simulink model "dynamic_model_dab"  (R2022b)
settings: Solver=VariableStepAuto  StartTime=0.0  StopTime=6.5e-2  RelTol=1e-3
libraries: spsMosfetLib x8, spsSeriesRLCBranchLib x5, spsEdgeDetectorLib x4, spsCurrentMeasurementLib x3, spsStairGeneratorLib x3, spsControlledVoltageSourceLib x2, spsMultimeterLib x2, spsLinearTransformerLib x1, eeGeneralControl x1, spsMeanVariableFrequencyLib x1, spsMeanLib x1, slpidlib x1
settings Model: Creator=srikr  LastModifiedBy=Pratik

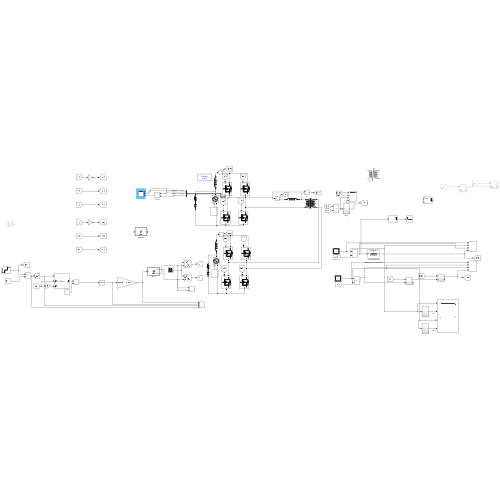
[thumbnail: Simulink's stored preview of the top-level diagram]
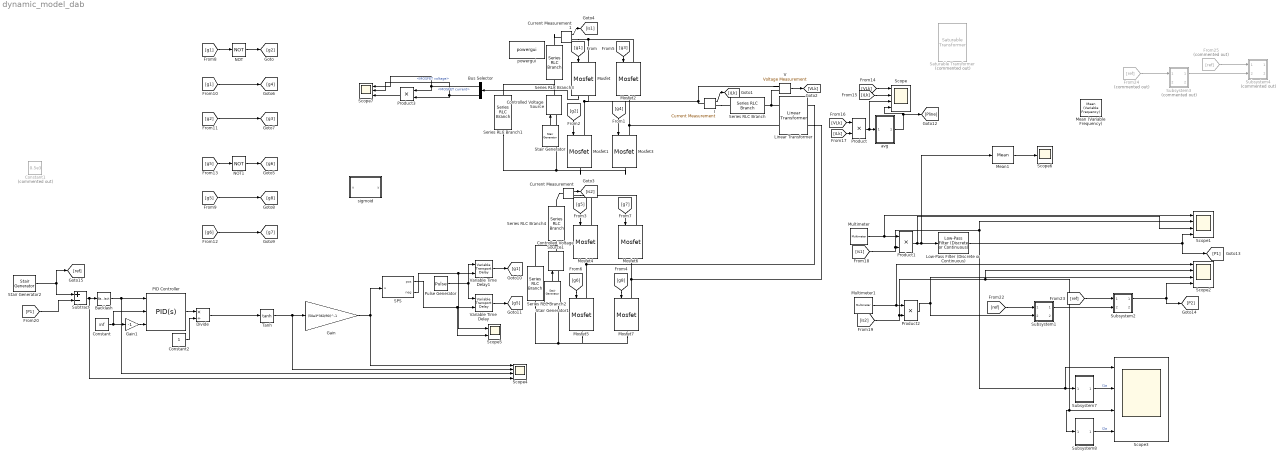
== system dynamic_model_dab ==
  Backlash : Backlash  BacklashWidth=0
  Bus Selector : BusSelector  OutputSignals=MOSFET current,MOSFET voltage
  Constant : Constant  Value=inf
  Constant1 : Constant  Commented=on  Value=0.5e3
  Constant2 : Constant
  Controlled Voltage Source : spsControlledVoltageSourceLib/Controlled Voltage Source  Initialize=on  Source_Type=AC  Amplitude=0  Phase=0  Frequency=0  Measurements=Voltage
  Controlled Voltage Source1 : spsControlledVoltageSourceLib/Controlled Voltage Source  Initialize=on  Source_Type=AC  Amplitude=0  Phase=0  Frequency=0  Measurements=Voltage
  Current Measurement : spsCurrentMeasurementLib/Current Measurement  PhasorSimulation=off  OutputType=Complex  PSBequivalent=0
  Current Measurement1 : spsCurrentMeasurementLib/Current Measurement  PhasorSimulation=off  OutputType=Complex  PSBequivalent=0
  Divide : Product  Inputs=*/
  From24 : From  Commented=on  GotoTag=ref
  From25 : From  Commented=on  GotoTag=ref
  Gain : Gain  Gain=(50e3*360/90)^-1
  Gain1 : Gain  Gain=-1
  I : spsCurrentMeasurementLib/Current Measurement  PhasorSimulation=off  OutputType=Complex  PSBequivalent=0
  Linear Transformer : spsLinearTransformerLib/Linear Transformer  UNITS=SI  NominalPower=[ 250e6 30e3 ]  winding1=[200 0 0]  winding2=[100 0 0]  ThreeWindings=off  winding3=[3.15e+05 0.7938 0.084225]  RmLm=[30e3 1e-3]  Measurements=All voltages and currents  DataType=on
  Low-Pass Filter (Discrete or Continuous) : eeGeneralControl/Low-Pass Filter (Discrete or Continuous)  K=1  T=1e-3  B=inf  A=-inf  init_option=Inherited from block input  x0=0  Ts=-1
  Mean (Variable Frequency) : spsMeanVariableFrequencyLib/Mean (Variable Frequency)  Finit=60  Fmin=45  Vinit=0  Ts=0
      settings: LibrarySourceBlock=|
      | sps_lib/Sensors and Measurements/Mean
      | (Variable Frequency)
  Mean1 : spsMeanLib/Mean  Freq=50e3  Vinit=0  Ts=0
  Mosfet : spsMosfetLib/Mosfet  Ron=0.1  Lon=0  Rd=0.01  Vfd=0  IC=0  Rs=1e5  Cs=inf  Measurements=on
  Mosfet{1..7} (7 alike) : spsMosfetLib/Mosfet  Ron=0.1  Lon=0  Rd=0.01  Vfd=0  IC=0  Rs=1e5  Cs=inf  Measurements=off
  Multimeter : spsMultimeterLib/Multimeter  L=11  sel=4  yselected={}  Gain=1  OutputType=Complex  PlotAtSimulationStop=off  PhasorSimulation=off
  Multimeter1 : spsMultimeterLib/Multimeter  L=11  sel=4  yselected={}  Gain=1  OutputType=Complex  PlotAtSimulationStop=off  PhasorSimulation=off
  NOT : Logic  Operator=NOT  IconShape=distinctive  AllPortsSameDT=off  OutDataTypeStr=boolean
  NOT1 : Logic  Operator=NOT  IconShape=distinctive  AllPortsSameDT=off  OutDataTypeStr=boolean
  PID Controller : slpidlib/PID Controller  Controller=PID  Form=Parallel  TimeDomain=Continuous-time  UseExternalTs=off  SampleTime=-1  IntegratorMethod=Forward Euler  FilterMethod=Forward Euler  ControllerParametersSource=internal  P=9e-2  I=0  UseKiTs=off  D=0  N=100  UseFilter=on  TunerSelectOption=Transfer Function Based (PID Tuner App)  InitialConditionSource=internal  InitialConditionForIntegrator=0  InitialConditionForFilter=0  DifferentiatorICPrevScaledInput=0  ExternalReset=none  TrackingMode=off  Kt=1  LimitOutput=on  SatLimitsSource=external  UpperSaturationLimit=1e3  LowerSaturationLimit=-1e3  LinearizeAsGain=on  AntiWindupMode=none  Kb=1  LimitIntegrator=off  UpperIntegratorSaturationLimit=inf  LowerIntegratorSaturationLimit=-inf  POutMin=[]  POutMax=[]  IOutMin=[]  IOutMax=[]  DOutMin=[]  DOutMax=[]  NOutMin=[]  NOutMax=[]  SumOutMin=[]  SumOutMax=[]  SaturationOutMin=[]  SaturationOutMax=[]  PParamMin=[]  PParamMax=[]  IParamMin=[]  IParamMax=[]  DParamMin=[]  DParamMax=[]  NParamMin=[]  NParamMax=[]  KbParamMin=[]  KbParamMax=[]  KtParamMin=[]  KtParamMax=[]  KbOutMin=[]  KbOutMax=[]  KtOutMin=[]  KtOutMax=[]  IntegratorOutMin=[]  IntegratorOutMax=[]  FilterOutMin=[]  FilterOutMax=[]  SumI1OutMin=[]  SumI1OutMax=[]  SumI2OutMin=[]  SumI2OutMax=[]  SumI3OutMin=[]  SumI3OutMax=[]  SumI4OutMin=[]  SumI4OutMax=[]  SumDOutMin=[]  SumDOutMax=[]  DifferentiatorOutMin=[]  DifferentiatorOutMax=[]  FilterDiffOutCoefMin=[]  FilterDiffOutCoefMax=[]  ReciprocalOutMin=[]  ReciprocalOutMax=[]  SumDenOutMin=[]  SumDenOutMax=[]  SumNumOutMin=[]  SumNumOutMax=[]  DivideOutMin=[]  DivideOutMax=[]  UdiffTsProdOutMin=[]  UdiffTsProdOutMax=[]  NTsProdOutMin=[]  NTsProdOutMax=[]  UintegralTsProdOutMin=[]  UintegralTsProdOutMax=[]  UngainTsProdOutMin=[]  UngainTsProdOutMax=[]  ClampingZeroOutDataTypeStr=Inherit: Inherit via back propagation  ClampingZeroOutMin=[]  ClampingZeroOutMax=[]  FilterDenConstantOutDataTypeStr=Inherit: Inherit via back propagation  FilterDenConstantOutMin=[]  FilterDenConstantOutMax=[]  PCopyOutDataTypeStr=Inherit: Inherit via back propagation  PCopyOutMin=[]  PCopyOutMax=[]  NCopyOutDataTypeStr=Inherit: Inherit via back propagation  NCopyOutMin=[]  NCopyOutMax=[]  IntegratorContinuousStateAttributes=''  IntegratorStateMustResolveToSignalObject=off  IntegratorRTWStateStorageClass=Auto  FilterContinuousStateAttributes=''  FilterStateMustResolveToSignalObject=off  FilterRTWStateStorageClass=Auto  ParallelPVariant=InternalParameters  IdealPVariant=Disabled  IVariant=InternalParameters  DVariant=InternalParameters  IntegratorVariant=Continuous  SatVariant=External  AWVariant=Passthrough  PCopyVariant=Disabled  TRVariant=Disabled  FdbkBlocksVariant=Forward  IdealPFdbkVariant=Disabled  SatFdbkVariant=Disabled  DerivativeFilterVariant=ContFilter  NVariant=InternalParameters  NCopyVariant=Disabled  FilterICVariant=InternalICsFilter  IntegratorICVariant=InternalICs  ExternalResetVariant=Disabled  TRSumVariant=Passthrough  SumFdbkVariant=Disabled  SumVariant=Sum_PID  TsampFilterVariant=InternalTs  TsampNgainVariant=Passthrough  TsampIntegralVariant=Passthrough  ExternalSaturationOutDataTypeStr=Inherit: Same as second input
  Product{,1..3} (4 alike) : Product
  Pulse Generator : DiscretePulseGenerator  PulseType=Time based  Period=1/50e3  PulseWidth=50
  SPS : MATLAB Function  TreatAsAtomicUnit=on
  Saturable Transformer : spsSaturableTransformerLib/Saturable Transformer  Commented=on  ThreeWindings=off  Hysteresis=off  DataFile='hysteresis.mat'  Measurements=All measurements (V I Flux)  UNITS=SI  NominalPower=[250e6 60]  Winding1=[200 0 0]  Winding2=[100 0 0]  Winding3=[3.15e+05 0.7938 0.084225]  Saturation=[0 0;1 100;]  CoreLoss=25e3  BreakLoop=off  DiscreteSolver=Trapezoidal iterative  DataType=on  InitialFlux=0  TransfoNumber=1
      settings: LibrarySourceBlock=sps_lib/Power Grid Elements/Saturable Transformer
  Scope{,1..4} (5 alike) : Scope  NumInputPorts=4
  Scope5 : Scope  NumInputPorts=2
  Scope6 : Scope
  Scope7 : Scope  NumInputPorts=3
  Series RLC Branch : spsSeriesRLCBranchLib/Series RLC Branch  LConnTagsString=__new0  RConnTagsString=__new0  BranchType=L  Resistance=1  Inductance=10e-6  SetiL0=off  InitialCurrent=0  Capacitance=1e-6  Setx0=off  InitialVoltage=0  Measurements=Branch voltage and current
  Series RLC Branch1 : spsSeriesRLCBranchLib/Series RLC Branch  LConnTagsString=__new0  RConnTagsString=__new0  BranchType=RC  Resistance=1e-9  Inductance=1e-3  SetiL0=off  InitialCurrent=0  Capacitance=1e-6  Setx0=off  InitialVoltage=0  Measurements=None
  Series RLC Branch2 : spsSeriesRLCBranchLib/Series RLC Branch  LConnTagsString=__new0  RConnTagsString=__new0  BranchType=RC  Resistance=1e-9  Inductance=1e-3  SetiL0=off  InitialCurrent=0  Capacitance=1e-6  Setx0=off  InitialVoltage=0  Measurements=None
  Series RLC Branch3 : spsSeriesRLCBranchLib/Series RLC Branch  LConnTagsString=__new0  RConnTagsString=__new0  BranchType=L  Resistance=1e-9  Inductance=2e-6  SetiL0=off  InitialCurrent=0  Capacitance=1e-9  Setx0=off  InitialVoltage=0  Measurements=None
  Series RLC Branch4 : spsSeriesRLCBranchLib/Series RLC Branch  LConnTagsString=__new0  RConnTagsString=__new0  BranchType=L  Resistance=1e-9  Inductance=2e-6  SetiL0=off  InitialCurrent=0  Capacitance=1e-9  Setx0=off  InitialVoltage=0  Measurements=None
  Stair Generator : spsStairGeneratorLib/Stair Generator  t=[0,0.5]*5e-2  e=[100, 100]  Ts=0
  Stair Generator1 : spsStairGeneratorLib/Stair Generator  t=[0,0.25]*5e-2  e=[100, 100]  Ts=0
  Stair Generator2 : spsStairGeneratorLib/Stair Generator  t=[0:.25:1]*5e-2  e=[0.5e3,-1e3,-0e3,1e3,0.5e3]  Ts=0
  Subsystem1 : Subsystem
  Subsystem2 : Subsystem
  Subsystem3 : Subsystem  Commented=on
  Subsystem4 : Subsystem  Commented=on
  Subsystem7 : Subsystem
  Subsystem8 : Subsystem
  Subtract : Sum  Inputs=+-
  Tanh : Trigonometry  Operator=tanh
  V : spsVoltageMeasurementLib/Voltage Measurement  PhasorSimulation=off  OutputType=Complex  PSBequivalent=0
  Variable Time Delay : VariableTransportDelay  MaximumDelay=10
  Variable Time Delay1 : VariableTransportDelay  MaximumDelay=10
  avg : Subsystem
  powergui : sps_lib/powergui  Priority=1  SimulationMode=Discrete  SampleTime=1e-6  frequency=60  Iterations=50  frequencyindice=0  Pbase=100e6  ErrMax=1e-4  UnitsV=kV  UnitsW=MW  buscounter=0  FunctionMessages=off  echomessages=off  EnableUseOfTLC=off  CurrentSourceSwitches=off  DisableSnubberDevices=off  DisableRonSwitches=off  DisableVfSwitches=off  DisplayEquations=off  AutomaticDiscreteSolvers=off  SolverType=Tustin/Backward Euler (TBE)  Interpol=off  ExternalGateDelay=off  methode=off  Ts=100  x0status=blocks  SPID=on  SwTol=0  HookPort=off  NonlinearTolerance=1e-4  nMaxIteration=100  ContinueOnMaxIteration=off  RestoreLinks=warning  ResistiveCurrentMeasurement=off  Frange=[0:2:500]  Ylog=off  Xlog=on  ShowGrid=off  save=off  variable=ZData  structure=0  ZoomFFT=off  StartTime=0.0  cycles=1  DisplayStyle=1  fundamental=60  FreqAxis=off  MaxFrequency=1000  frequencyindicesteady=1  RmsSteady=1  display=off
  sigmoid : MATLAB Function  TreatAsAtomicUnit=on
  wires:
  [g8] -> Mosfet7/1
  [g1] -> NOT/1
  NOT/1 -> [g2]
  [g1] -> [g4]
  [g2] -> [g3]
  [g5] -> NOT1/1
  [g5] -> [g8]
  [g6] -> [g7]
  NOT1/1 -> [g6]
  Pulse Generator/1 -> Variable Time Delay1/1, Variable Time Delay/1
  Variable Time Delay/1 -> [g5]
  Gain/1 -> SPS/1(u), Scope4/1
  I/1 -> [iLk]
  V/1 -> [VLk]
  [VLk] -> Scope/1
  [iLk] -> Scope/2
  Product/1 -> Scope/3, avg/1(In1)
  [VLk] -> Product/1
  [iLk] -> Product/2
  avg/1(Out1) -> [Pline], Scope/4
  Current Measurement/1 -> [is2]
  Multimeter/1 -> Product1/1, Scope1/1
  [is1] -> Scope3/1, Subsystem7/1(In1), Scope1/2, Product1/2
  Current Measurement1/1 -> [is1]
  [is2] -> Subsystem8/1(In1), Scope3/3, Scope2/2, Product2/2
  Multimeter1/1 -> Product2/1, Scope2/1
  Stair Generator/1 -> Controlled Voltage Source/1
  Subsystem7/1(Out1) -> Scope3/2  "I1a"
  Subsystem8/1(Out1) -> Scope3/4  "I2a"
  Stair Generator1/1 -> Controlled Voltage Source1/1
  Subtract/1 -> Scope4/4, Backlash/1
  Stair Generator2/1 -> Subtract/1, [ref]
  [P1] -> Subtract/2
  Subsystem2/1(Out1) -> [P2], Scope2/4
  Variable Time Delay1/1 -> [g1]
  Backlash/1 -> Scope4/3, PID Controller/1
  Constant/1 -> PID Controller/2, Gain1/1
  Gain1/1 -> PID Controller/3
  PID Controller/1 -> Divide/1
  Constant2/1 -> Divide/2
  Tanh/1 -> Gain/1, Scope4/2
  Product2/1 -> Scope2/3, Subsystem1/2(In2)
  [ref] -> Subsystem1/1(In1)
  Subsystem1/1(Out1) -> Subsystem2/2(In2)
  [ref] -> Subsystem2/1(In1)
  Subsystem3/1(Out1) -> Subsystem4/2(In2)
  From25/1 -> Subsystem4/1(In1)
  From24/1 -> Subsystem3/1(In1)
  Product1/1 -> Low-Pass Filter (Discrete or Continuous)/1, Mean1/1, Scope1/3
  SPS/1(pos) -> Scope5/2, Variable Time Delay/2
  SPS/2(neg) -> Scope5/1, Variable Time Delay1/2
  Mean1/1 -> Scope6/1
  Low-Pass Filter (Discrete or Continuous)/1 -> [P1], Scope1/4
  [g1] -> Mosfet/1
  [g2] -> Mosfet1/1
  [g4] -> Mosfet3/1
  [g3] -> Mosfet2/1
  [g5] -> Mosfet4/1
  [g6] -> Mosfet5/1
  [g7] -> Mosfet6/1
  Divide/1 -> Tanh/1
  Bus Selector/1 -> Scope7/1, Product3/1  "<MOSFET current>"
  Mosfet/1 -> Bus Selector/1
  Bus Selector/2 -> Scope7/2, Product3/2  "<MOSFET voltage>"
  Product3/1 -> Scope7/3
  connections:
  Current Measurement1/RConn1 -- Mosfet/LConn1 -- Mosfet2/LConn1
  Series RLC Branch1/RConn1 -- Controlled Voltage Source/LConn1 -- Mosfet3/RConn1 -- Mosfet1/RConn1
  Series RLC Branch2/RConn1 -- Mosfet7/RConn1 -- Mosfet5/RConn1 -- Controlled Voltage Source1/LConn1
  Current Measurement/RConn1 -- Mosfet4/LConn1 -- Mosfet6/LConn1
  Series RLC Branch/RConn1 -- V/LConn2 -- Linear Transformer/LConn1
  I/RConn1 -- Series RLC Branch/LConn1
  Controlled Voltage Source/RConn1 -- Series RLC Branch1/LConn1 -- Series RLC Branch3/RConn1
  Series RLC Branch4/LConn1 -- Current Measurement/LConn1
  I/LConn1 -- V/LConn1 -- Mosfet1/LConn1 -- Mosfet/RConn1
  Mosfet3/LConn1 -- Mosfet2/RConn1 -- Linear Transformer/LConn2
  Mosfet4/RConn1 -- Linear Transformer/RConn1 -- Mosfet5/LConn1
  Mosfet7/LConn1 -- Mosfet6/RConn1 -- Linear Transformer/RConn2
  Series RLC Branch3/LConn1 -- Current Measurement1/LConn1
  Controlled Voltage Source1/RConn1 -- Series RLC Branch2/LConn1 -- Series RLC Branch4/RConn1

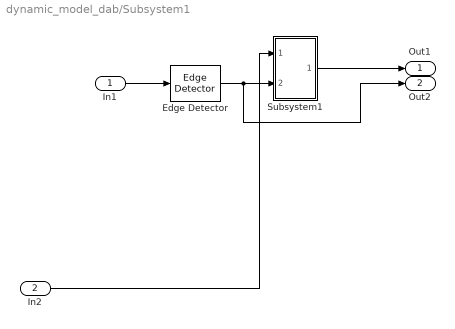
== system dynamic_model_dab/Subsystem1 ==
  In1 : Inport
  In2 : Inport  Port=2
  Edge Detector : spsEdgeDetectorLib/Edge Detector  model=Either  ic=0  Ts=0
      settings: LibrarySourceBlock=sps_lib/Control/Edge Detector
  Subsystem1 : Subsystem
  Out1 : Outport
  Out2 : Outport  Port=2
  wires:
  Edge Detector/1 -> Out2/1, Subsystem1/2(Input)
  Subsystem1/1(Out1) -> Out1/1
  In1/1 -> Edge Detector/1
  In2/1 -> Subsystem1/1(In1)

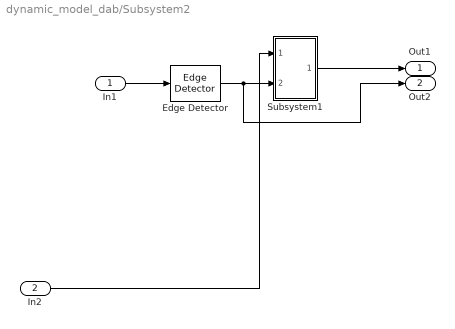
== system dynamic_model_dab/Subsystem2 ==
  In1 : Inport
  In2 : Inport  Port=2
  Edge Detector : spsEdgeDetectorLib/Edge Detector  model=Either  ic=0  Ts=0
      settings: LibrarySourceBlock=sps_lib/Control/Edge Detector
  Subsystem1 : Subsystem
  Out1 : Outport
  Out2 : Outport  Port=2
  wires:
  Edge Detector/1 -> Out2/1, Subsystem1/2(Input)
  Subsystem1/1(Out1) -> Out1/1
  In1/1 -> Edge Detector/1
  In2/1 -> Subsystem1/1(In1)

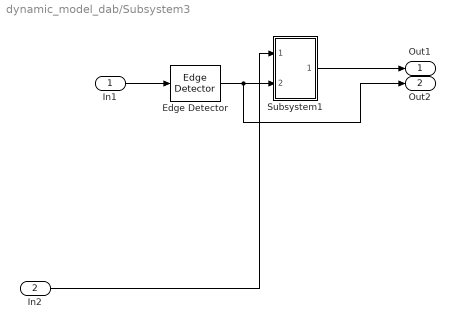
== system dynamic_model_dab/Subsystem3 ==
  In1 : Inport
  In2 : Inport  Port=2
  Edge Detector : spsEdgeDetectorLib/Edge Detector  model=Either  ic=0  Ts=0
      settings: LibrarySourceBlock=sps_lib/Control/Edge Detector
  Subsystem1 : Subsystem
  Out1 : Outport
  Out2 : Outport  Port=2
  wires:
  Edge Detector/1 -> Out2/1, Subsystem1/2(Input)
  Subsystem1/1(Out1) -> Out1/1
  In1/1 -> Edge Detector/1
  In2/1 -> Subsystem1/1(In1)

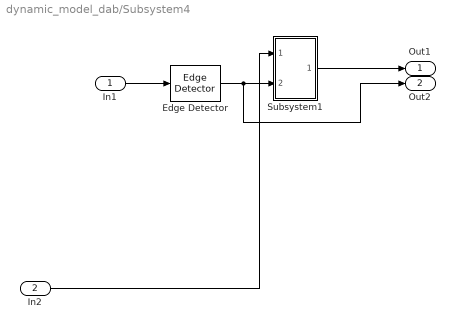
== system dynamic_model_dab/Subsystem4 ==
  In1 : Inport
  In2 : Inport  Port=2
  Edge Detector : spsEdgeDetectorLib/Edge Detector  model=Either  ic=0  Ts=0
      settings: LibrarySourceBlock=sps_lib/Control/Edge Detector
  Subsystem1 : Subsystem
  Out1 : Outport
  Out2 : Outport  Port=2
  wires:
  Edge Detector/1 -> Out2/1, Subsystem1/2(Input)
  Subsystem1/1(Out1) -> Out1/1
  In1/1 -> Edge Detector/1
  In2/1 -> Subsystem1/1(In1)

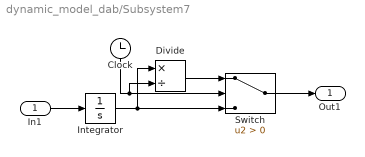
== system dynamic_model_dab/Subsystem7 ==
  In1 : Inport
  Clock : Clock
  Divide : Product  Inputs=*/
  Integrator : Integrator
  Switch : Switch  Criteria=u2 > Threshold  SaturateOnIntegerOverflow=off  InputSameDT=off
  Out1 : Outport
  wires:
  Divide/1 -> Switch/1
  Integrator/1 -> Switch/3, Divide/1
  Clock/1 -> Switch/2, Divide/2
  In1/1 -> Integrator/1
  Switch/1 -> Out1/1

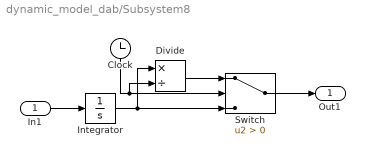
== system dynamic_model_dab/Subsystem8 ==
  In1 : Inport
  Clock : Clock
  Divide : Product  Inputs=*/
  Integrator : Integrator
  Switch : Switch  Criteria=u2 > Threshold  SaturateOnIntegerOverflow=off  InputSameDT=off
  Out1 : Outport
  wires:
  Divide/1 -> Switch/1
  Integrator/1 -> Switch/3, Divide/1
  Clock/1 -> Switch/2, Divide/2
  In1/1 -> Integrator/1
  Switch/1 -> Out1/1

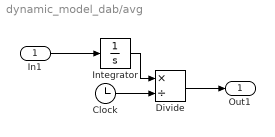
== system dynamic_model_dab/avg ==
  In1 : Inport
  Clock : Clock
  Divide : Product  Inputs=*/
  Integrator : Integrator
  Out1 : Outport
  wires:
  Divide/1 -> Out1/1
  Clock/1 -> Divide/2
  Integrator/1 -> Divide/1
  In1/1 -> Integrator/1

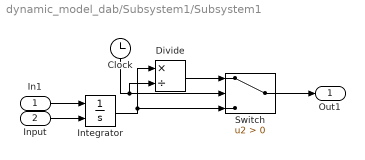
== system dynamic_model_dab/Subsystem1/Subsystem1 ==
  In1 : Inport
  Input : Inport  Port=2
  Clock : Clock
  Divide : Product  Inputs=*/
  Integrator : Integrator  ExternalReset=rising  LimitOutput=on  IgnoreLimit=on
  Switch : Switch  Criteria=u2 > Threshold  SaturateOnIntegerOverflow=off  InputSameDT=off
  Out1 : Outport
  wires:
  Divide/1 -> Switch/1
  Integrator/1 -> Switch/3, Divide/1
  Clock/1 -> Switch/2, Divide/2
  In1/1 -> Integrator/1
  Switch/1 -> Out1/1
  Input/1 -> Integrator/2

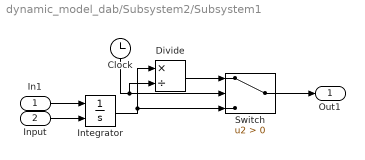
== system dynamic_model_dab/Subsystem2/Subsystem1 ==
  In1 : Inport
  Input : Inport  Port=2
  Clock : Clock
  Divide : Product  Inputs=*/
  Integrator : Integrator  ExternalReset=rising  LimitOutput=on  IgnoreLimit=on
  Switch : Switch  Criteria=u2 > Threshold  SaturateOnIntegerOverflow=off  InputSameDT=off
  Out1 : Outport
  wires:
  Divide/1 -> Switch/1
  Integrator/1 -> Switch/3, Divide/1
  Clock/1 -> Switch/2, Divide/2
  In1/1 -> Integrator/1
  Switch/1 -> Out1/1
  Input/1 -> Integrator/2

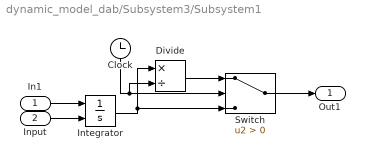
== system dynamic_model_dab/Subsystem3/Subsystem1 ==
  In1 : Inport
  Input : Inport  Port=2
  Clock : Clock
  Divide : Product  Inputs=*/
  Integrator : Integrator  ExternalReset=rising  LimitOutput=on  IgnoreLimit=on
  Switch : Switch  Criteria=u2 > Threshold  SaturateOnIntegerOverflow=off  InputSameDT=off
  Out1 : Outport
  wires:
  Divide/1 -> Switch/1
  Integrator/1 -> Switch/3, Divide/1
  Clock/1 -> Switch/2, Divide/2
  In1/1 -> Integrator/1
  Switch/1 -> Out1/1
  Input/1 -> Integrator/2

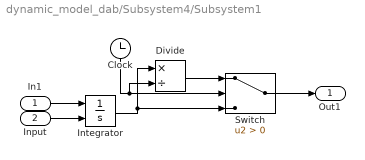
== system dynamic_model_dab/Subsystem4/Subsystem1 ==
  In1 : Inport
  Input : Inport  Port=2
  Clock : Clock
  Divide : Product  Inputs=*/
  Integrator : Integrator  ExternalReset=rising  LimitOutput=on  IgnoreLimit=on
  Switch : Switch  Criteria=u2 > Threshold  SaturateOnIntegerOverflow=off  InputSameDT=off
  Out1 : Outport
  wires:
  Divide/1 -> Switch/1
  Integrator/1 -> Switch/3, Divide/1
  Clock/1 -> Switch/2, Divide/2
  In1/1 -> Integrator/1
  Switch/1 -> Out1/1
  Input/1 -> Integrator/2

== matlab function dynamic_model_dab/sigmoid ==
  data: u input; y output
function y = fcn(u)

y = 1/(1 + exp(-u));

== matlab function dynamic_model_dab/SPS ==
  data: u input; pos output; neg output
function [pos,neg] = fcn(u)

if u>=0
    pos = u;
    neg = 0;
else
    neg = -u;
    pos = 0;
end
